simulink model "QFTmodel"  (R2020a)
settings: Solver=FixedStepAuto  StartTime=0.0  StopTime=20.0  FixedStep=0.07053  RelTol=1e-3  EnableMultiTasking=on
values from neighbouring files (symbols this model uses):
  Ay = A(1)    [QFT_Controller_Design.m]
  Tau = T(1)    [QFT_Controller_Design.m]
undefined symbols (not defined in the file or in its folder): DiscIntNeverNeededParam
libraries: simulink_extras x1
settings Model: Creator=User  LastModifiedBy=Daniel
settings DataIOCC: ReturnWorkspaceOutputs=off
settings OptimizationCC: LifeSpan=inf
settings DebuggingCC: SFUnexpectedBacktrackingDiag=warning  SFNoUnconditionalDefaultTransitionDiag=warning  ArithmeticOperatorsInVariantConditions=warning
settings SFSimCC: SimUseLocalCustomCode=off  CustomCodeUndefinedFunction=UseInterfaceOnly
settings RTWCC: RTWUseLocalCustomCode=off
settings CodeAppCC: StateflowObjectComments=on
settings GRTTargetCC: TargetLangStandard=C89/C90 (ANSI)
settings ConfigComp: CovMetricSettings=dw  CovHtmlReporting=on  CovSaveCumulativeToWorkspaceVar=on  CovSaveSingleToWorkspaceVar=on  CovExternalEMLEnable=off

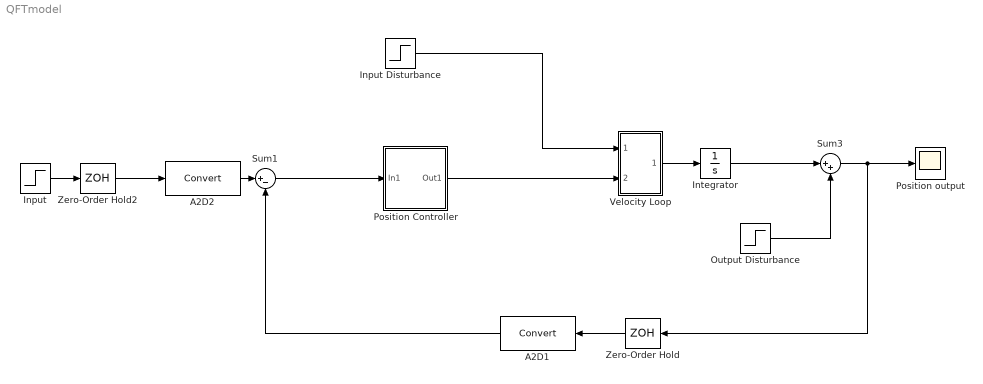
== system QFTmodel ==
  A2D1 : DataTypeConversion
  A2D2 : DataTypeConversion
  Input : Step  Time=0  SampleTime=0
  Input Disturbance : Step  Time=8  SampleTime=0
  Integrator : Integrator
  Output Disturbance : Step  Time=14  SampleTime=0
  Position Controller : Subsystem
  Position output : Scope
  Sum1 : Sum  Inputs=|+-
  Sum3 : Sum  Inputs=|++
  Velocity Loop : Subsystem
  Zero-Order Hold : ZeroOrderHold  SampleTime=-1
  Zero-Order Hold2 : ZeroOrderHold  SampleTime=-1
  wires:
  Output Disturbance/1 -> Sum3/2
  Sum3/1 -> Zero-Order Hold/1, Position output/1
  Sum1/1 -> Position Controller/1(In1)
  A2D1/1 -> Sum1/2
  Zero-Order Hold/1 -> A2D1/1
  Zero-Order Hold2/1 -> A2D2/1
  A2D2/1 -> Sum1/1
  Input/1 -> Zero-Order Hold2/1
  Input Disturbance/1 -> Velocity Loop/1(In1)
  Position Controller/1(Out1) -> Velocity Loop/2(In2)
  Velocity Loop/1(Out1) -> Integrator/1
  Integrator/1 -> Sum3/1

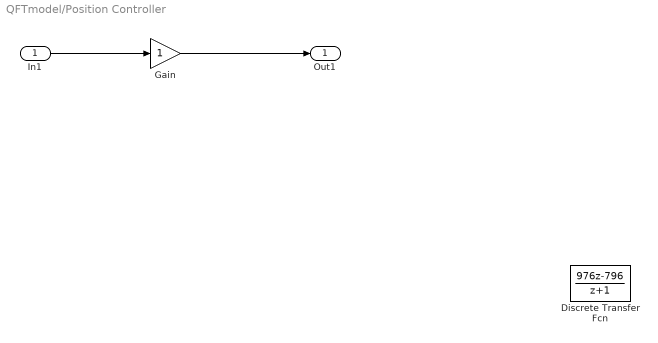
== system QFTmodel/Position Controller ==
  In1 : Inport
  Discrete Transfer Fcn : DiscreteTransferFcn  Numerator=[976 -796]  Denominator=[1 1]
  Gain : Gain
  Out1 : Outport
  wires:
  In1/1 -> Gain/1
  Gain/1 -> Out1/1

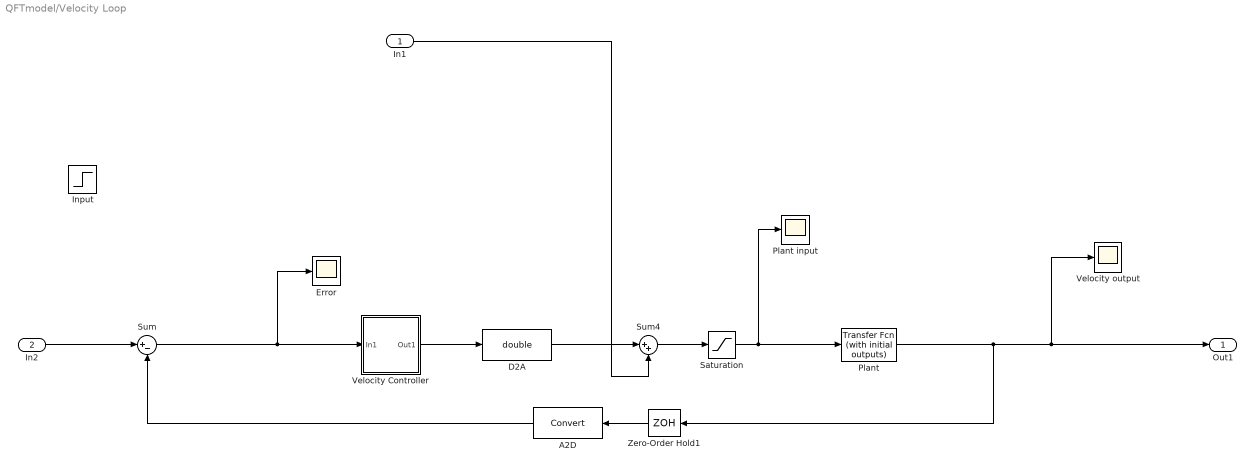
== system QFTmodel/Velocity Loop ==
  In1 : Inport
  In2 : Inport  Port=2
  " Saturation" : Saturate  UpperLimit=10  LowerLimit=-10
  A2D : DataTypeConversion
  D2A : DataTypeConversion  OutDataTypeStr=double
  Error : Scope
  Input : Step  Time=0  SampleTime=0
  Plant : simulink_extras/Additional Linear/Transfer Fcn (with initial outputs)  N=[Ay]  D="[1  Tau]"  Y0=0  U0=0
  Plant input : Scope
  Sum : Sum  Inputs=|+-
  Sum4 : Sum  Inputs=|++
  Velocity Controller : Subsystem
  Velocity output : Scope
  Zero-Order Hold1 : ZeroOrderHold  SampleTime=-1
  Out1 : Outport
  wires:
  Sum4/1 -> " Saturation"/1
  Plant/1 -> Out1/1, Velocity output/1, Zero-Order Hold1/1
  A2D/1 -> Sum/2
  Velocity Controller/1(Out1) -> D2A/1
  Sum/1 -> Velocity Controller/1(In1), Error/1
  Zero-Order Hold1/1 -> A2D/1
  " Saturation"/1 -> Plant input/1, Plant/1
  In1/1 -> Sum4/2
  D2A/1 -> Sum4/1
  In2/1 -> Sum/1

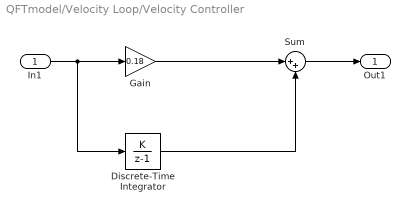
== system QFTmodel/Velocity Loop/Velocity Controller ==
  In1 : Inport
  Discrete-Time Integrator : DiscreteIntegrator  IntegratorMethod=Accumulation: Forward Euler  gainval=0.08  SampleTime=-1  ICPrevOutput=DiscIntNeverNeededParam  ICPrevScaledInput=DiscIntNeverNeededParam
  Gain : Gain  Gain=0.18
  Sum : Sum  Inputs=|++
  Out1 : Outport
  wires:
  Sum/1 -> Out1/1
  In1/1 -> Discrete-Time Integrator/1, Gain/1
  Gain/1 -> Sum/1
  Discrete-Time Integrator/1 -> Sum/2
